simulink model "ball_balancing_omni3_multibody_lqi"  (R2026a)
settings: Solver=ode15s  StopTime=ballbotParams.simulation.stopTime  MaxStep=ballbotParams.simulation.maxStep  RelTol=ballbotParams.simulation.relativeTolerance
PreLoadFcn:
  | ballbotParams = ballbotParameters;
undefined symbols (not defined in the file or in its folder): ballbotEstimatorInitialState, ballbotEstimatorUpdate, ballbotImuFromJoint, ballbotLqiControllerUpdate, ballbotPoseFromJoint, ballbotServoVoltageController, ballbotWheelRateFromDisplacement, X, Y, Z
libraries: nesl_utility x38, sm_lib x26, fl_lib x12, ee_lib x3
(part 3 of 3)

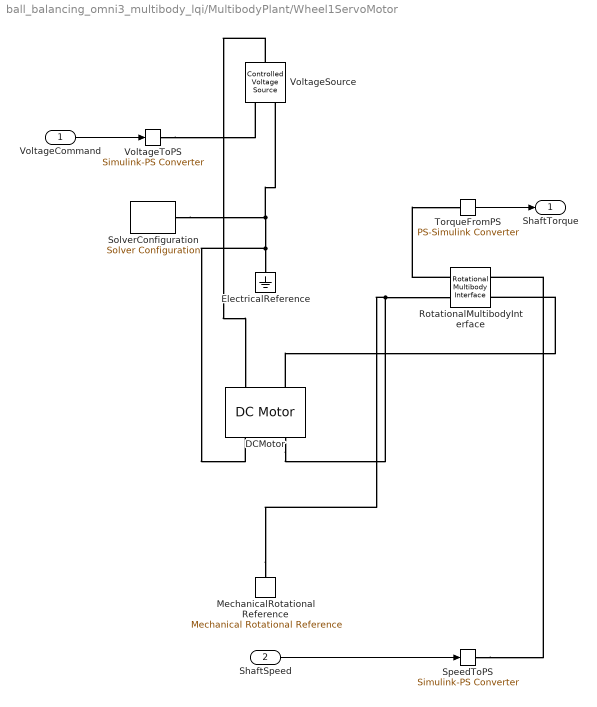
== system ball_balancing_omni3_multibody_lqi/MultibodyPlant/Wheel1ServoMotor ==
  VoltageCommand : Inport
  ShaftSpeed : Inport  Port=2
  DCMotor : ee_lib/Electromechanical/Brushed Motors/DC Motor  field_option=ee.enum.field_option.pm  Rf=100 Ohm  Lf=1 H  Laf=0.15 H  If0=0 A  parameterization=ee.enum.dcparam_option.torque_speed  Ra=3.9 Ohm  La=12e-6 H  emf_or_torque=ee.enum.emf_or_torque.kv  Kv=0.072e-3 V/rpm  Ki=6.876e-4 N*m/A  T_stall=ballbotParams.servo.maxTorque N*m  w_max=ballbotParams.servo.maxSpeed rpm  w_rated=15000 rpm  P_rated=0.08 W  V_rated=ballbotParams.servo.nominalVoltage V  lam_param=ee.enum.lam_param.damping  i_noload=ballbotParams.servo.operatingCurrent A  V_i_noload=1.5 V  J=ballbotParams.servo.equivalentInertia cm^2*g  lam=0 N*m*s/rad  speed0=0 rpm  alpha=3.93e-3 1/K  Tmeas=25 degC  thermal_mass=100 J/K  initial_temperature=25 degC
  ElectricalReference : fl_lib/Electrical/Electrical Elements/Electrical Reference
  MechanicalRotationalReference : fl_lib/Mechanical/Rotational Elements/Mechanical Rotational Reference
  RotationalMultibodyInterface : fl_lib/Mechanical/Multibody Interfaces/Rotational Multibody Interface
  SolverConfiguration : nesl_utility/Solver Configuration  PhysicalDomain=network_engine_domain  SubClassName=solver  LeftPortType=input  RightPortType=generic  Tones=[]  Harmonics=[]  SimulateNoise=off  Profile=off  UseLocalSampling=off  EnableSwitchedLinearOptims=on  FrequencyDomain=off  UseCCode=off  RelTol=0.001  AbsTol=0.001  MinStep=1e-09  ToWorkspace=off  RevertToSquareIcSolve=off  NumHomotopyIterations=100  PhasorMode=off  PhasorModeNumHarmonics=1  ConsistencySolver=NEWTON_XTOL_AFTER_FTOL  CanonicalOrdering=CANONICAL  OptimizeIntermediates=OPTIMIZED  IndexReductionMethod=DerivativeReplacement  DoDC=off  ResidualTolerance=1e-09  ConsistencyTolSource=GLOBAL  ConsistencyAbsTol=0.001  ConsistencyRelTol=0.001  ConsistencyTolFactor=0.001  UseLocalSolver=off  LocalSolverChoice=NE_BACKWARD_EULER_ADVANCER  ResolveIndetEquations=on  FunctionEvalNumThread=1  LocalSolverSampleTime=0.001  DoFixedCost=off  MaxNonlinIter=3  MaxModeIter=2  ComputeImpulses=off  ImpulseIterations=2  LinearAlgebra=auto  LinearAlgebraNumThread=0  EquationFormulation=NE_TIME_EF  DelaysMemoryBudget=1024  AutomaticFiltering=on  FilteringTimeConstant=0.001  PartitionStorageMethod=AS_NEEDED  PartitionMemoryBudget=1024  PartitionMethod=ROBUST  MultibodyUseLocalSolver=off  MultibodyLocalSolverChoice=ODE1  MultibodyLocalSolverSampleTime=0.001
  SpeedToPS : nesl_utility/Simulink-PS Converter  PhysicalDomain=network_engine_domain  SubClassName=ps_input  LeftPortType=input  RightPortType=output  PseudoPeriodic=off  Frequencies=[]  NoiseDistribution=none  NoiseParameters=[]  Unit=rad/s  AffineConversion=off  FilteringAndDerivatives=filter  SimscapeFilterOrder=1  InputFilterTimeConstant=1e-4  UdotUserProvided=0
  TorqueFromPS : nesl_utility/PS-Simulink Converter  PhysicalDomain=network_engine_domain  SubClassName=ps_output  LeftPortType=input  RightPortType=output  PseudoPeriodic=off  Frequencies=[]  VectorFormat=inherit  Unit=N*m  AffineConversion=off
  VoltageSource : fl_lib/Electrical/Electrical Sources/Controlled Voltage Source
  VoltageToPS : nesl_utility/Simulink-PS Converter  PhysicalDomain=network_engine_domain  SubClassName=ps_input  LeftPortType=input  RightPortType=output  PseudoPeriodic=off  Frequencies=[]  NoiseDistribution=none  NoiseParameters=[]  Unit=V  AffineConversion=off  FilteringAndDerivatives=provide  SimscapeFilterOrder=1  InputFilterTimeConstant=0.001  UdotUserProvided=0
  ShaftTorque : Outport
  wires:
  VoltageCommand/1 -> VoltageToPS/1
  ShaftSpeed/1 -> SpeedToPS/1
  TorqueFromPS/1 -> ShaftTorque/1
  connections:
  RotationalMultibodyInterface/LConn1 -- TorqueFromPS/LConn1
  SpeedToPS/RConn1 -- RotationalMultibodyInterface/RConn1
  VoltageToPS/RConn1 -- VoltageSource/RConn1
  VoltageSource/LConn1 -- DCMotor/LConn1
  VoltageSource/RConn2 -- ElectricalReference/LConn1 -- DCMotor/RConn1 -- SolverConfiguration/RConn1
  DCMotor/LConn2 -- RotationalMultibodyInterface/RConn2
  MechanicalRotationalReference/LConn1 -- RotationalMultibodyInterface/LConn2 -- DCMotor/RConn2

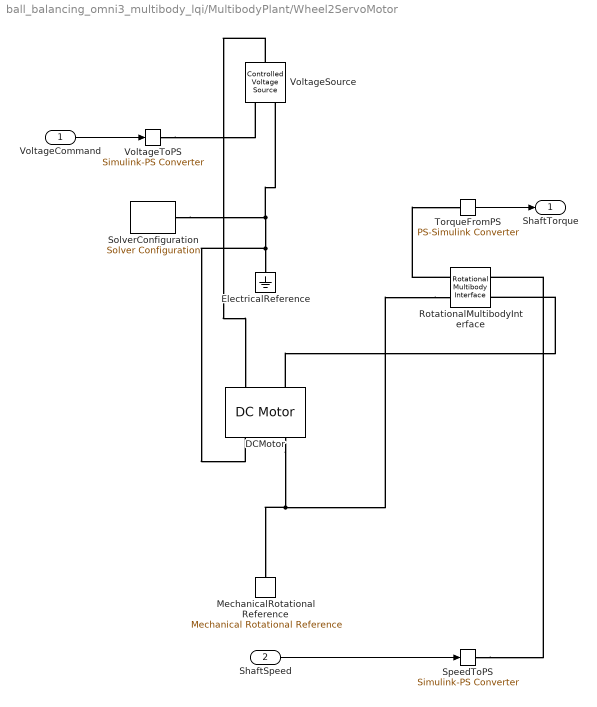
== system ball_balancing_omni3_multibody_lqi/MultibodyPlant/Wheel2ServoMotor ==
  VoltageCommand : Inport
  ShaftSpeed : Inport  Port=2
  DCMotor : ee_lib/Electromechanical/Brushed Motors/DC Motor  field_option=ee.enum.field_option.pm  Rf=100 Ohm  Lf=1 H  Laf=0.15 H  If0=0 A  parameterization=ee.enum.dcparam_option.torque_speed  Ra=3.9 Ohm  La=12e-6 H  emf_or_torque=ee.enum.emf_or_torque.kv  Kv=0.072e-3 V/rpm  Ki=6.876e-4 N*m/A  T_stall=ballbotParams.servo.maxTorque N*m  w_max=ballbotParams.servo.maxSpeed rpm  w_rated=15000 rpm  P_rated=0.08 W  V_rated=ballbotParams.servo.nominalVoltage V  lam_param=ee.enum.lam_param.damping  i_noload=ballbotParams.servo.operatingCurrent A  V_i_noload=1.5 V  J=ballbotParams.servo.equivalentInertia cm^2*g  lam=0 N*m*s/rad  speed0=0 rpm  alpha=3.93e-3 1/K  Tmeas=25 degC  thermal_mass=100 J/K  initial_temperature=25 degC
  ElectricalReference : fl_lib/Electrical/Electrical Elements/Electrical Reference
  MechanicalRotationalReference : fl_lib/Mechanical/Rotational Elements/Mechanical Rotational Reference
  RotationalMultibodyInterface : fl_lib/Mechanical/Multibody Interfaces/Rotational Multibody Interface
  SolverConfiguration : nesl_utility/Solver Configuration  PhysicalDomain=network_engine_domain  SubClassName=solver  LeftPortType=input  RightPortType=generic  Tones=[]  Harmonics=[]  SimulateNoise=off  Profile=off  UseLocalSampling=off  EnableSwitchedLinearOptims=on  FrequencyDomain=off  UseCCode=off  RelTol=0.001  AbsTol=0.001  MinStep=1e-09  ToWorkspace=off  RevertToSquareIcSolve=off  NumHomotopyIterations=100  PhasorMode=off  PhasorModeNumHarmonics=1  ConsistencySolver=NEWTON_XTOL_AFTER_FTOL  CanonicalOrdering=CANONICAL  OptimizeIntermediates=OPTIMIZED  IndexReductionMethod=DerivativeReplacement  DoDC=off  ResidualTolerance=1e-09  ConsistencyTolSource=GLOBAL  ConsistencyAbsTol=0.001  ConsistencyRelTol=0.001  ConsistencyTolFactor=0.001  UseLocalSolver=off  LocalSolverChoice=NE_BACKWARD_EULER_ADVANCER  ResolveIndetEquations=on  FunctionEvalNumThread=1  LocalSolverSampleTime=0.001  DoFixedCost=off  MaxNonlinIter=3  MaxModeIter=2  ComputeImpulses=off  ImpulseIterations=2  LinearAlgebra=auto  LinearAlgebraNumThread=0  EquationFormulation=NE_TIME_EF  DelaysMemoryBudget=1024  AutomaticFiltering=on  FilteringTimeConstant=0.001  PartitionStorageMethod=AS_NEEDED  PartitionMemoryBudget=1024  PartitionMethod=ROBUST  MultibodyUseLocalSolver=off  MultibodyLocalSolverChoice=ODE1  MultibodyLocalSolverSampleTime=0.001
  SpeedToPS : nesl_utility/Simulink-PS Converter  PhysicalDomain=network_engine_domain  SubClassName=ps_input  LeftPortType=input  RightPortType=output  PseudoPeriodic=off  Frequencies=[]  NoiseDistribution=none  NoiseParameters=[]  Unit=rad/s  AffineConversion=off  FilteringAndDerivatives=filter  SimscapeFilterOrder=1  InputFilterTimeConstant=1e-4  UdotUserProvided=0
  TorqueFromPS : nesl_utility/PS-Simulink Converter  PhysicalDomain=network_engine_domain  SubClassName=ps_output  LeftPortType=input  RightPortType=output  PseudoPeriodic=off  Frequencies=[]  VectorFormat=inherit  Unit=N*m  AffineConversion=off
  VoltageSource : fl_lib/Electrical/Electrical Sources/Controlled Voltage Source
  VoltageToPS : nesl_utility/Simulink-PS Converter  PhysicalDomain=network_engine_domain  SubClassName=ps_input  LeftPortType=input  RightPortType=output  PseudoPeriodic=off  Frequencies=[]  NoiseDistribution=none  NoiseParameters=[]  Unit=V  AffineConversion=off  FilteringAndDerivatives=provide  SimscapeFilterOrder=1  InputFilterTimeConstant=0.001  UdotUserProvided=0
  ShaftTorque : Outport
  wires:
  TorqueFromPS/1 -> ShaftTorque/1
  ShaftSpeed/1 -> SpeedToPS/1
  VoltageCommand/1 -> VoltageToPS/1
  connections:
  RotationalMultibodyInterface/LConn2 -- MechanicalRotationalReference/LConn1 -- DCMotor/RConn2
  DCMotor/LConn2 -- RotationalMultibodyInterface/RConn2
  DCMotor/RConn1 -- SolverConfiguration/RConn1 -- VoltageSource/RConn2 -- ElectricalReference/LConn1
  VoltageSource/LConn1 -- DCMotor/LConn1
  RotationalMultibodyInterface/LConn1 -- TorqueFromPS/LConn1
  SpeedToPS/RConn1 -- RotationalMultibodyInterface/RConn1
  VoltageToPS/RConn1 -- VoltageSource/RConn1

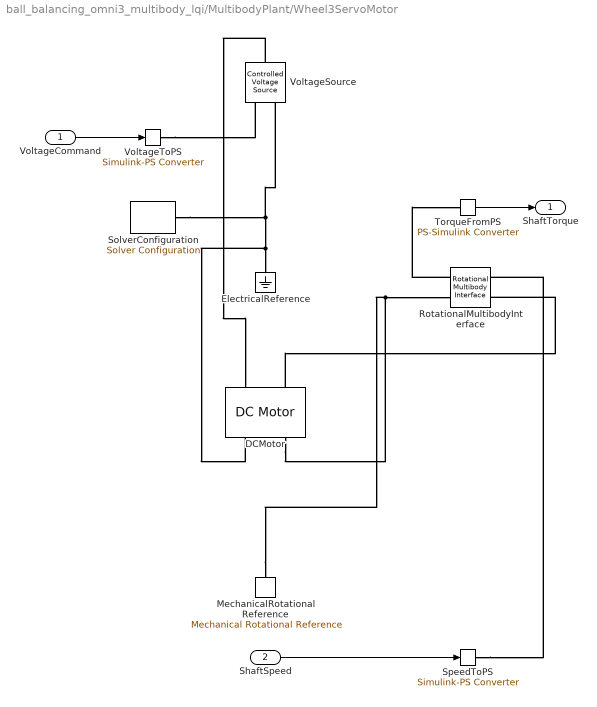
== system ball_balancing_omni3_multibody_lqi/MultibodyPlant/Wheel3ServoMotor ==
  VoltageCommand : Inport
  ShaftSpeed : Inport  Port=2
  DCMotor : ee_lib/Electromechanical/Brushed Motors/DC Motor  field_option=ee.enum.field_option.pm  Rf=100 Ohm  Lf=1 H  Laf=0.15 H  If0=0 A  parameterization=ee.enum.dcparam_option.torque_speed  Ra=3.9 Ohm  La=12e-6 H  emf_or_torque=ee.enum.emf_or_torque.kv  Kv=0.072e-3 V/rpm  Ki=6.876e-4 N*m/A  T_stall=ballbotParams.servo.maxTorque N*m  w_max=ballbotParams.servo.maxSpeed rpm  w_rated=15000 rpm  P_rated=0.08 W  V_rated=ballbotParams.servo.nominalVoltage V  lam_param=ee.enum.lam_param.damping  i_noload=ballbotParams.servo.operatingCurrent A  V_i_noload=1.5 V  J=ballbotParams.servo.equivalentInertia cm^2*g  lam=0 N*m*s/rad  speed0=0 rpm  alpha=3.93e-3 1/K  Tmeas=25 degC  thermal_mass=100 J/K  initial_temperature=25 degC
  ElectricalReference : fl_lib/Electrical/Electrical Elements/Electrical Reference
  MechanicalRotationalReference : fl_lib/Mechanical/Rotational Elements/Mechanical Rotational Reference
  RotationalMultibodyInterface : fl_lib/Mechanical/Multibody Interfaces/Rotational Multibody Interface
  SolverConfiguration : nesl_utility/Solver Configuration  PhysicalDomain=network_engine_domain  SubClassName=solver  LeftPortType=input  RightPortType=generic  Tones=[]  Harmonics=[]  SimulateNoise=off  Profile=off  UseLocalSampling=off  EnableSwitchedLinearOptims=on  FrequencyDomain=off  UseCCode=off  RelTol=0.001  AbsTol=0.001  MinStep=1e-09  ToWorkspace=off  RevertToSquareIcSolve=off  NumHomotopyIterations=100  PhasorMode=off  PhasorModeNumHarmonics=1  ConsistencySolver=NEWTON_XTOL_AFTER_FTOL  CanonicalOrdering=CANONICAL  OptimizeIntermediates=OPTIMIZED  IndexReductionMethod=DerivativeReplacement  DoDC=off  ResidualTolerance=1e-09  ConsistencyTolSource=GLOBAL  ConsistencyAbsTol=0.001  ConsistencyRelTol=0.001  ConsistencyTolFactor=0.001  UseLocalSolver=off  LocalSolverChoice=NE_BACKWARD_EULER_ADVANCER  ResolveIndetEquations=on  FunctionEvalNumThread=1  LocalSolverSampleTime=0.001  DoFixedCost=off  MaxNonlinIter=3  MaxModeIter=2  ComputeImpulses=off  ImpulseIterations=2  LinearAlgebra=auto  LinearAlgebraNumThread=0  EquationFormulation=NE_TIME_EF  DelaysMemoryBudget=1024  AutomaticFiltering=on  FilteringTimeConstant=0.001  PartitionStorageMethod=AS_NEEDED  PartitionMemoryBudget=1024  PartitionMethod=ROBUST  MultibodyUseLocalSolver=off  MultibodyLocalSolverChoice=ODE1  MultibodyLocalSolverSampleTime=0.001
  SpeedToPS : nesl_utility/Simulink-PS Converter  PhysicalDomain=network_engine_domain  SubClassName=ps_input  LeftPortType=input  RightPortType=output  PseudoPeriodic=off  Frequencies=[]  NoiseDistribution=none  NoiseParameters=[]  Unit=rad/s  AffineConversion=off  FilteringAndDerivatives=filter  SimscapeFilterOrder=1  InputFilterTimeConstant=1e-4  UdotUserProvided=0
  TorqueFromPS : nesl_utility/PS-Simulink Converter  PhysicalDomain=network_engine_domain  SubClassName=ps_output  LeftPortType=input  RightPortType=output  PseudoPeriodic=off  Frequencies=[]  VectorFormat=inherit  Unit=N*m  AffineConversion=off
  VoltageSource : fl_lib/Electrical/Electrical Sources/Controlled Voltage Source
  VoltageToPS : nesl_utility/Simulink-PS Converter  PhysicalDomain=network_engine_domain  SubClassName=ps_input  LeftPortType=input  RightPortType=output  PseudoPeriodic=off  Frequencies=[]  NoiseDistribution=none  NoiseParameters=[]  Unit=V  AffineConversion=off  FilteringAndDerivatives=provide  SimscapeFilterOrder=1  InputFilterTimeConstant=0.001  UdotUserProvided=0
  ShaftTorque : Outport
  wires:
  TorqueFromPS/1 -> ShaftTorque/1
  ShaftSpeed/1 -> SpeedToPS/1
  VoltageCommand/1 -> VoltageToPS/1
  connections:
  MechanicalRotationalReference/LConn1 -- RotationalMultibodyInterface/LConn2 -- DCMotor/RConn2
  DCMotor/LConn2 -- RotationalMultibodyInterface/RConn2
  DCMotor/RConn1 -- SolverConfiguration/RConn1 -- VoltageSource/RConn2 -- ElectricalReference/LConn1
  VoltageSource/LConn1 -- DCMotor/LConn1
  RotationalMultibodyInterface/LConn1 -- TorqueFromPS/LConn1
  SpeedToPS/RConn1 -- RotationalMultibodyInterface/RConn1
  VoltageToPS/RConn1 -- VoltageSource/RConn1
